simulink model "OMAP"  (R2018b)
settings: Solver=FixedStepDiscrete  StartTime=0.0  StopTime=10.0  FixedStep=0.01  RelTol=1e-3
values from neighbouring files (symbols this model uses):
  Clb_ICADirect_LaneDisp_StateFive = Simulink.Parameter    [omap_ver_442.m]
  Clb_ICADirect_LaneDisp_StateFour = Simulink.Parameter    [omap_ver_442.m]
  Clb_ICADirect_LaneDisp_StateOne = Simulink.Parameter    [omap_ver_442.m]
  Clb_ICADirect_LaneDisp_StateThree = Simulink.Parameter    [omap_ver_442.m]
  Clb_ICADirect_LaneDisp_StateTwo = Simulink.Parameter    [omap_ver_442.m]
  Clb_ICADirect_LaneDisp_StateZero = Simulink.Parameter    [omap_ver_442.m]
  Clb_ICADirect_LaneDispSW = Simulink.Parameter    [omap_ver_442.m]
  Clb_ICADirect_TrnLghtsCom_Switch = Simulink.Parameter    [omap_ver_442.m]
  Clb_ICADirect_TrnLghtsCom_Value = Simulink.Parameter    [omap_ver_442.m]
  Clb_ICADirect_TrnLghtsCrtl_Inhb = Simulink.Parameter    [omap_ver_442.m]
  OMAP_ACCAEB_EMSESC_Decel = Simulink.Parameter    [omap_ver_442.m]
  OMAP_ACCFCW_IC_Decel = Simulink.Parameter    [omap_ver_442.m]
  OMAP_clb_ACC_RVVReqType = Simulink.Parameter    [omap_ver_442.m]
  OMAP_clb_ACC_RVVReqType_Switch = Simulink.Parameter    [omap_ver_442.m]
  OMAP_clb_ACCHeadwayDisplay = Simulink.Parameter    [omap_ver_442.m]
  OMAP_clb_ACCHeadwayDisplay_Switch = Simulink.Parameter    [omap_ver_442.m]
  OMAP_clb_ACCHeadwayIcon = Simulink.Parameter    [omap_ver_442.m]
  OMAP_clb_ACCHeadwayIcon_Switch = Simulink.Parameter    [omap_ver_442.m]
  OMAP_clb_ACCMessagePrompt = Simulink.Parameter    [omap_ver_442.m]
  OMAP_clb_ACCMessagePrompt_Switch = Simulink.Parameter    [omap_ver_442.m]
  OMAP_clb_ACCRequestEPB = Simulink.Parameter    [omap_ver_442.m]
  OMAP_clb_ACCRequestEPB_Switch = Simulink.Parameter    [omap_ver_442.m]
  OMAP_clb_ACCSetSpeed = Simulink.Parameter    [omap_ver_442.m]
  OMAP_clb_ACCSetSpeed_Switch = Simulink.Parameter    [omap_ver_442.m]
  OMAP_clb_ACCSetSpeedDis = Simulink.Parameter    [omap_ver_442.m]
  OMAP_clb_ACCSetSpeedDis_Switch = Simulink.Parameter    [omap_ver_442.m]
  OMAP_clb_ACCState = Simulink.Parameter    [omap_ver_442.m]
  OMAP_clb_ACCState_Switch = Simulink.Parameter    [omap_ver_442.m]
  OMAP_clb_ACCStatusIconDis = Simulink.Parameter    [omap_ver_442.m]
  OMAP_clb_ACCStatusIconDis_Switch = Simulink.Parameter    [omap_ver_442.m]
  OMAP_clb_ACCTorqueReq = Simulink.Parameter    [omap_ver_442.m]
  OMAP_clb_ACCTorqueReq_Switch = Simulink.Parameter    [omap_ver_442.m]
  OMAP_clb_ADAS_State = Simulink.Parameter    [omap_ver_442.m]
  OMAP_clb_ADAS_State_Switch = Simulink.Parameter    [omap_ver_442.m]
  OMAP_clb_AEBAlertReq = Simulink.Parameter    [omap_ver_442.m]
  OMAP_clb_AEBAlertReq_Switch = Simulink.Parameter    [omap_ver_442.m]
  OMAP_clb_AEBBrakingProg = Simulink.Parameter    [omap_ver_442.m]
  OMAP_clb_AEBBrakingProg_Switch = Simulink.Parameter    [omap_ver_442.m]
  OMAP_clb_AEBFaultStatus = Simulink.Parameter    [omap_ver_442.m]
  OMAP_clb_AEBFaultStatus_Switch = Simulink.Parameter    [omap_ver_442.m]
  OMAP_clb_AEBMassageDisp = Simulink.Parameter    [omap_ver_442.m]
  OMAP_clb_AEBMassageDisp_Switch = Simulink.Parameter    [omap_ver_442.m]
  OMAP_clb_AEBState = Simulink.Parameter    [omap_ver_442.m]
  OMAP_clb_AEBState_Switch = Simulink.Parameter    [omap_ver_442.m]
  OMAP_clb_AEBSwitchStatus = Simulink.Parameter    [omap_ver_442.m]
  OMAP_clb_AEBSwitchStatus_Switch = Simulink.Parameter    [omap_ver_442.m]
  OMAP_clb_BrakeRequest = Simulink.Parameter    [omap_ver_442.m]
  OMAP_clb_BrakeRequest_Switch = Simulink.Parameter    [omap_ver_442.m]
  OMAP_clb_DecelerationSet = Simulink.Parameter    [omap_ver_442.m]
  OMAP_clb_DecelerationSet_Switch = Simulink.Parameter    [omap_ver_442.m]
  OMAP_clb_DecelerationType = Simulink.Parameter    [omap_ver_442.m]
  OMAP_clb_DecelerationType_Switch = Simulink.Parameter    [omap_ver_442.m]
  OMAP_clb_DeclControlReq = Simulink.Parameter    [omap_ver_442.m]
  OMAP_clb_DeclControlReq_Switch = Simulink.Parameter    [omap_ver_442.m]
  OMAP_clb_DownorUpGearMinTime = Simulink.Parameter    [omap_ver_442.m]
  OMAP_clb_DownorUpGearMinTime_Switch = Simulink.Parameter    [omap_ver_442.m]
  OMAP_clb_ELKPopupMessage = Simulink.Parameter    [omap_ver_442.m]
  OMAP_clb_ELKPopupMessage_Switch = Simulink.Parameter    [omap_ver_442.m]
  OMAP_clb_ELKSts = Simulink.Parameter    [omap_ver_442.m]
  OMAP_clb_ELKSts_Switch = Simulink.Parameter    [omap_ver_442.m]
  OMAP_clb_ESAFaultSt = Simulink.Parameter    [omap_ver_442.m]
  OMAP_clb_ESAFaultSt_Switch = Simulink.Parameter    [omap_ver_442.m]
  OMAP_clb_ESARequest = Simulink.Parameter    [omap_ver_442.m]
  OMAP_clb_ESARequest_Switch = Simulink.Parameter    [omap_ver_442.m]
  OMAP_clb_ESAState = Simulink.Parameter    [omap_ver_442.m]
  OMAP_clb_ESAState_Switch = Simulink.Parameter    [omap_ver_442.m]
  OMAP_clb_ESATorqueReq = Simulink.Parameter    [omap_ver_442.m]
  OMAP_clb_ESATorqueReq_Switch = Simulink.Parameter    [omap_ver_442.m]
  OMAP_clb_ESCDriveOff = Simulink.Parameter    [omap_ver_442.m]
  OMAP_clb_ESCDriveOff_Switch = Simulink.Parameter    [omap_ver_442.m]
  OMAP_clb_ESCHoldReq = Simulink.Parameter    [omap_ver_442.m]
  OMAP_clb_ESCHoldReq_Switch = Simulink.Parameter    [omap_ver_442.m]
  OMAP_clb_Handsoffwarning = Simulink.Parameter    [omap_ver_442.m]
  OMAP_clb_Handsoffwarning_Switch = Simulink.Parameter    [omap_ver_442.m]
  OMAP_clb_HapticAlarmReq = Simulink.Parameter    [omap_ver_442.m]
  OMAP_clb_HapticAlarmReq_Switch = Simulink.Parameter    [omap_ver_442.m]
  OMAP_clb_HMIPopupMassage = Simulink.Parameter    [omap_ver_442.m]
  OMAP_clb_HMIPopupMassage_Switch = Simulink.Parameter    [omap_ver_442.m]
  OMAP_clb_HWAActionSts = Simulink.Parameter    [omap_ver_442.m]
  OMAP_clb_HWAActionSts_Switch = Simulink.Parameter    [omap_ver_442.m]
  OMAP_clb_HWAMode = Simulink.Parameter    [omap_ver_442.m]
  OMAP_clb_HWAMode_Switch = Simulink.Parameter    [omap_ver_442.m]
  OMAP_clb_HWATurnOnIdctr = Simulink.Parameter    [omap_ver_442.m]
  OMAP_clb_HWATurnOnIdctr_Switch = Simulink.Parameter    [omap_ver_442.m]
  OMAP_clb_ICAMassageDisp = Simulink.Parameter    [omap_ver_442.m]
  OMAP_clb_ICAMassageDisp_Switch = Simulink.Parameter    [omap_ver_442.m]
  OMAP_clb_ICAStatusIcon = Simulink.Parameter    [omap_ver_442.m]
  OMAP_clb_ICAStatusIcon_Switch = Simulink.Parameter    [omap_ver_442.m]
  OMAP_clb_ISLCDriverRemind = Simulink.Parameter    [omap_ver_442.m]
  OMAP_clb_ISLCDriverRemind_Switch = Simulink.Parameter    [omap_ver_442.m]
  OMAP_clb_ISLCState = Simulink.Parameter    [omap_ver_442.m]
  OMAP_clb_ISLCState_Switch = Simulink.Parameter    [omap_ver_442.m]
  OMAP_clb_JAFaultSt = Simulink.Parameter    [omap_ver_442.m]
  OMAP_clb_JAFaultSt_Switch = Simulink.Parameter    [omap_ver_442.m]
  OMAP_clb_LCAPopupMessage = Simulink.Parameter    [omap_ver_442.m]
  OMAP_clb_LCAPopupMessage_Switch = Simulink.Parameter    [omap_ver_442.m]
  OMAP_clb_LCAStatusDisplay = Simulink.Parameter    [omap_ver_442.m]
  OMAP_clb_LCAStatusDisplay_Switch = Simulink.Parameter    [omap_ver_442.m]
  OMAP_clb_LDWStatusDisplay = Simulink.Parameter    [omap_ver_442.m]
  OMAP_clb_LDWStatusDisplay_Switch = Simulink.Parameter    [omap_ver_442.m]
  OMAP_clb_LDWWarningSt = Simulink.Parameter    [omap_ver_442.m]
  OMAP_clb_LDWWarningSt_Switch = Simulink.Parameter    [omap_ver_442.m]
  OMAP_clb_LightControlValid = Simulink.Parameter    [omap_ver_442.m]
  OMAP_clb_LightControlValid_Switch = Simulink.Parameter    [omap_ver_442.m]
  OMAP_clb_LKAActivation = Simulink.Parameter    [omap_ver_442.m]
  OMAP_clb_LKAActivation_Switch = Simulink.Parameter    [omap_ver_442.m]
  OMAP_clb_LKAAngleReq = Simulink.Parameter    [omap_ver_442.m]
  OMAP_clb_LKAAngleReq_Switch = Simulink.Parameter    [omap_ver_442.m]
  OMAP_clb_LKAMode = Simulink.Parameter    [omap_ver_442.m]
  OMAP_clb_LKAMode_Switch = Simulink.Parameter    [omap_ver_442.m]
  OMAP_clb_LKAorELK_CoolTime = Simulink.Parameter    [omap_ver_442.m]
  OMAP_clb_LKAState = Simulink.Parameter    [omap_ver_442.m]
  OMAP_clb_LKAState_Switch = Simulink.Parameter    [omap_ver_442.m]
  OMAP_clb_LKAStatusDisplay = Simulink.Parameter    [omap_ver_442.m]
  OMAP_clb_LKAStatusDisplay_Switch = Simulink.Parameter    [omap_ver_442.m]
  OMAP_clb_LKASwitchState = Simulink.Parameter    [omap_ver_442.m]
  OMAP_clb_LKASwitchState_Switch = Simulink.Parameter    [omap_ver_442.m]
  OMAP_clb_LKATorqFactReq = Simulink.Parameter    [omap_ver_442.m]
  OMAP_clb_LKATorqFactReq_Switch = Simulink.Parameter    [omap_ver_442.m]
  OMAP_clb_PrefillRequest = Simulink.Parameter    [omap_ver_442.m]
  ... (+36 more)
libraries: simulink x184, canmsglib x2
(part 4 of 14)

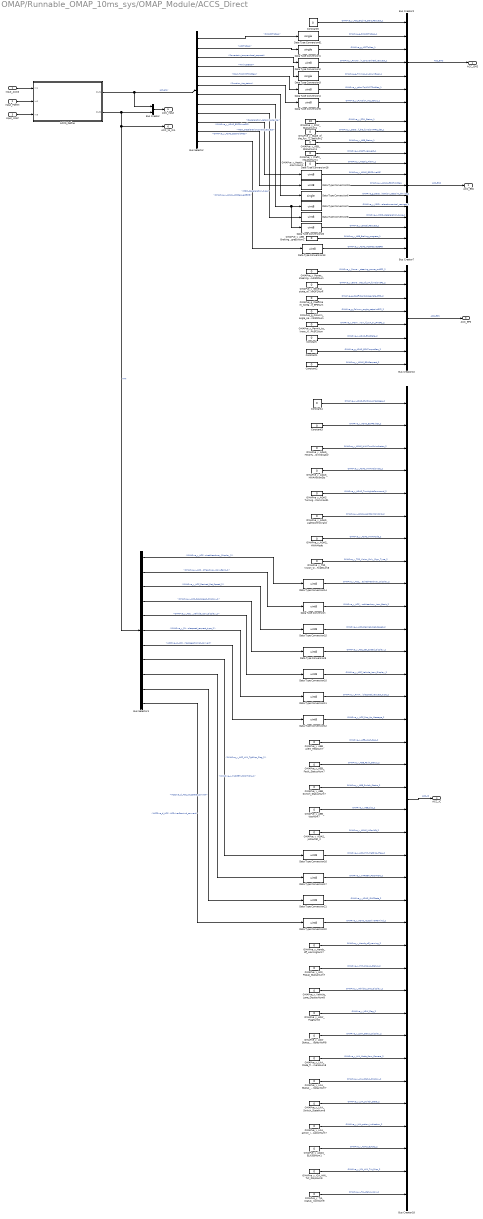
== system OMAP/Runnable_OMAP_10ms_sys/OMAP_Module/ACCS_Direct ==
  Input_ACCS : Inport
  Input_FDMM : Inport  Port=2
  Input_IMAP : Inport  Port=3
  ACCS_Define : Subsystem
  Bus Creator : BusCreator  Inputs=2
  Bus Creator10 : BusCreator  Inputs=8
  Bus Creator18 : BusCreator  Inputs=36
  Bus Creator2 : BusCreator  Inputs=7
  Bus Creator7 : BusCreator  Inputs=13
  Bus Selector : BusSelector  OutputSignals=PotACCTqReq,ACCTqReq,Powertrain_torquewheel_request,TminUpGear,StAcvTqWhlPTPotReq,Function_Acc_status,Deceleration_setpoint_device,MDD_Decelerationcontrol_request,MDD_deceleration_type,OMAPve_y_ADAS_ESCDriveOff,OMAPve_y_ADAS_ESCHoldReq,OMAPve_y_ADAS_ACCRequestEPB
  Bus Selector1 : BusSelector  OutputSignals=OMAPve_y_ACC_DesiredHeadway_Display_2,OMAPve_y_ACC_DesiredHeadway_Icon_Basic_2,OMAPve_y_ACC_Desired_Set_Speed_2,OMAPve_y_ACC_Set_Speed_Display_2,OMAPve_y_ACC_Vehicle_Icon_Display_2,OMAPve_y_RVVACC_Vehiclespeed_request_type_2,ACCSve_d_ACCMessagePrompt_convert,OMAPve_y_ACC_HMI_TgtDisp_Flag_2,OMAPve_y_TARGET_POSITION_2,ACCSve_d_ACC_ISLCState_convert,ACCSve_d_ACC_ISLCDriverRemind_convert
  Constant{,2..5} (5 alike) : Constant  Value=0  OutDataTypeStr=uint8
  Constant1 : Constant  Value=0  OutDataTypeStr=single
  Data Type Conversion{,2,4..5,7..22} (20 alike) : DataTypeConversion  OutDataTypeStr=uint8
  Data Type Conversion{1,3,6,61} (4 alike) : DataTypeConversion  OutDataTypeStr=single
  OMAPve_g_Coefficient_toregulate_EPSNum : Constant  Value=0  OutDataTypeStr=single
  OMAPve_g_Column_angle_setpoint3F2Num : Constant  Value=0  OutDataTypeStr=single
  OMAPve_y_ADAS_ELKStsNum1 : Constant  Value=0  OutDataTypeStr=uint8
  OMAPve_y_ADAS_HWAActionSts : Constant  Value=0  OutDataTypeStr=uint8
  OMAPve_y_ADAS_HWAMode : Constant  Value=0  OutDataTypeStr=uint8
  OMAPve_y_ADAS_HWATurnOnIndicator : Constant  Value=0  OutDataTypeStr=uint8
  OMAPve_y_ADAS_JAFaultSt_2 : Constant  Value=0  OutDataTypeStr=uint8
  OMAPve_y_ADAS_LightControlValid : Constant  Value=0  OutDataTypeStr=uint8
  OMAPve_y_ADAS_TurnLightsCommand1 : Constant  Value=0  OutDataTypeStr=uint8
  OMAPve_y_AEB_Alert_ReqNum7 : Constant  Value=0  OutDataTypeStr=uint8
  OMAPve_y_AEB_Braking_progressNum1 : Constant  Value=0  OutDataTypeStr=uint8
  OMAPve_y_AEB_Fault_StatusNum7 : Constant  Value=0  OutDataTypeStr=uint8
  OMAPve_y_AEB_StatusNum1 : Constant  Value=0  OutDataTypeStr=uint8
  OMAPve_y_AEB_Switch_StatusNum7 : Constant  Value=0  OutDataTypeStr=uint8
  OMAPve_y_AEB_tipsNum7 : Constant  Value=0  OutDataTypeStr=uint8
  OMAPve_y_FCW_StatusNum1 : Constant  Value=10  OutDataTypeStr=uint8
  OMAPve_y_General_state_of_LKA_function3F2Num : Constant  Value=0  OutDataTypeStr=uint8
  OMAPve_y_HMI_Popup_StatusNum7 : Constant  Value=0  OutDataTypeStr=uint8
  OMAPve_y_Hands_off_warningNum7 : Constant  Value=0  OutDataTypeStr=uint8
  OMAPve_y_Haptic_AlarmNum1 : Constant  Value=0  OutDataTypeStr=uint8
  OMAPve_y_ICA_HMI_Txt_DispNum9 : Constant  Value=0  OutDataTypeStr=uint8
  OMAPve_y_LDW_FlagNum8 : Constant  Value=0  OutDataTypeStr=uint8
  OMAPve_y_LDW_Status_DisplayNum8 : Constant  Value=0  OutDataTypeStr=uint8
  OMAPve_y_LKA_Mode_from_CameraNum8 : Constant  Value=0  OutDataTypeStr=uint8
  OMAPve_y_LKA_Status_DisplayNum7 : Constant  Value=0  OutDataTypeStr=uint8
  OMAPve_y_LKA_Switch_StateNum8 : Constant  Value=0  OutDataTypeStr=uint8
  OMAPve_y_LKA_action_indicationNum7 : Constant  Value=0  OutDataTypeStr=uint8
  OMAPve_y_Permit_to_know_if_LKA_or_LPA3F2Num : Constant  Value=0  OutDataTypeStr=uint8
  OMAPve_y_Power_steering_power_cut3F2Num : Constant  Value=0  OutDataTypeStr=uint8
  OMAPve_y_Prefill_requestNum1 : Constant  Value=0  OutDataTypeStr=uint8
  OMAPve_y_State_of_the_functionFARC_detNum1 : Constant  Value=0  OutDataTypeStr=uint8
  OMAPve_y_TJA_status_iconNum9 : Constant  Value=0  OutDataTypeStr=uint8
  OMAPve_y_TSR_Vision_Only_Sign_TypeNum8 : Constant  Value=0  OutDataTypeStr=uint8
  OMAPve_y_Vehicle_Lane_DisplayNum8 : Constant  Value=0  OutDataTypeStr=uint8
  ACC_EMS : Outport
  ACC_ESC : Outport  Port=2
  ACC_EPS : Outport  Port=3
  ACC_IC : Outport  Port=4
  ACC_Input : Outport  Port=5
  ACC_to_ICA : Outport  Port=6
  wires:
  Bus Selector/9 -> Data Type Conversion8/1  "<MDD_deceleration_type>"
  Bus Selector/8 -> Data Type Conversion20/1, Data Type Conversion7/1  "<MDD_Decelerationcontrol_request>"
  Bus Selector/7 -> Data Type Conversion6/1  "<Deceleration_setpoint_device>"
  Bus Selector/6 -> Data Type Conversion5/1  "<Function_Acc_status>"
  Bus Selector/5 -> Data Type Conversion4/1  "<StAcvTqWhlPTPotReq>"
  Bus Selector/4 -> Data Type Conversion3/1  "<TminUpGear>"
  Bus Selector/3 -> Data Type Conversion2/1  "<Powertrain_torquewheel_request>"
  Bus Selector/2 -> Data Type Conversion1/1  "<ACCTqReq>"
  Bus Selector/1 -> Data Type Conversion61/1  "<PotACCTqReq>"
  Input_FDMM/1 -> ACCS_Define/2(In2)
  Input_ACCS/1 -> ACCS_Define/1(In1)
  Bus Selector1/6 -> Data Type Conversion11/1  "<OMAPve_y_RVVACC_Vehiclespeed_request_type_2>"
  Bus Selector1/7 -> Data Type Conversion12/1  "<ACCSve_d_ACCMessagePrompt_convert>"
  Data Type Conversion1/1 -> Bus Creator2/3  "OMAPve_g_ACCTqReq_1"
  OMAPve_y_AEB_StatusNum1/1 -> Bus Creator7/3  "OMAPve_y_AEB_Status_1"
  Data Type Conversion6/1 -> Bus Creator7/8  "OMAPve_g_Deceleration_setpoint_device_1"
  Data Type Conversion8/1 -> Bus Creator7/10  "OMAPve_y_MDD_deceleration_type_1"
  Bus Selector1/5 -> Data Type Conversion10/1  "<OMAPve_y_ACC_Vehicle_Icon_Display_2>"
  Bus Creator18/1 -> ACC_IC/1  "ACC_IC"
  OMAPve_y_LDW_Status_DisplayNum8/1 -> Bus Creator18/29  "OMAPve_y_LDW_Status_Display_2"
  Bus Creator7/1 -> ACC_ESC/1  "ACC_ESC"
  OMAPve_y_AEB_tipsNum7/1 -> Bus Creator18/19  "OMAPve_y_AEB_tips_2"
  Bus Selector1/9 -> Data Type Conversion17/1  "<OMAPve_y_TARGET_POSITION_2>"
  Bus Selector1/3 -> Data Type Conversion15/1  "<OMAPve_y_ACC_Desired_Set_Speed_2>"
  Bus Selector1/1 -> Data Type Conversion14/1  "<OMAPve_y_ACC_DesiredHeadway_Display_2>"
  OMAPve_y_HMI_Popup_StatusNum7/1 -> Bus Creator18/26  "OMAPve_y_HMI_Popup_Status_2"
  OMAPve_y_AEB_Alert_ReqNum7/1 -> Bus Creator18/16  "OMAPve_y_AEB_Alert_Req_2"
  Bus Creator2/1 -> ACC_EMS/1  "ACC_EMS"
  OMAPve_y_TSR_Vision_Only_Sign_TypeNum8/1 -> Bus Creator18/8  "OMAPve_y_TSR_Vision_Only_Sign_Type_2"
  OMAPve_y_LDW_FlagNum8/1 -> Bus Creator18/28  "OMAPve_y_LDW_Flag_2"
  OMAPve_y_AEB_Fault_StatusNum7/1 -> Bus Creator18/17  "OMAPve_y_AEB_Fault_Status_2"
  OMAPve_y_State_of_the_functionFARC_detNum1/1 -> Bus Creator7/2  "OMAPve_y_State_of_the_functionFARC_det_1"
  OMAPve_y_Haptic_AlarmNum1/1 -> Bus Creator7/5  "OMAPve_y_Haptic_Alarm_1"
  OMAPve_y_ICA_HMI_Txt_DispNum9/1 -> Bus Creator18/35  "OMAPve_y_ICA_HMI_Txt_Disp_2"
  Data Type Conversion4/1 -> Bus Creator2/6  "OMAPve_y_stAcvTqWhlPTPotReq_1"
  Data Type Conversion20/1 -> Bus Creator7/11  "OMAPve_y_Decel_Request_1"
  Bus Selector1/2 -> Data Type Conversion/1  "<OMAPve_y_ACC_DesiredHeadway_Icon_Basic_2>"
  Data Type Conversion61/1 -> Bus Creator2/2  "OMAPve_g_PotACCTqReq_1"
  Bus Selector1/8 -> Data Type Conversion16/1  "<OMAPve_y_ACC_HMI_TgtDisp_Flag_2>"
  OMAPve_y_FCW_StatusNum1/1 -> Bus Creator7/1  "OMAPve_y_FCW_Status_1"
  OMAPve_y_Hands_off_warningNum7/1 -> Bus Creator18/25  "OMAPve_y_Hands_off_warning_2"
  OMAPve_y_AEB_Braking_progressNum1/1 -> Bus Creator7/12  "OMAPve_y_AEB_Braking_progress_1"
  Data Type Conversion5/1 -> Bus Creator2/7  "OMAPve_y_Function_Acc_status_1"
  OMAPve_y_LKA_Status_DisplayNum7/1 -> Bus Creator18/31  "OMAPve_y_LKA_Status_Display_2"
  Data Type Conversion3/1 -> Bus Creator2/5  "OMAPve_g_TminUp_or_downGear_1"
  OMAPve_y_Vehicle_Lane_DisplayNum8/1 -> Bus Creator18/27  "OMAPve_y_Vehicle_Lane_Display_2"
  OMAPve_y_AEB_Switch_StatusNum7/1 -> Bus Creator18/18  "OMAPve_y_AEB_Switch_Status_2"
  Constant5/1 -> Bus Creator2/1  "OMAPve_y_ACC_Engine_Start_Request_1"
  OMAPve_y_TJA_status_iconNum9/1 -> Bus Creator18/36  "OMAPve_y_TJA_status_icon_2"
  OMAPve_y_LKA_action_indicationNum7/1 -> Bus Creator18/33  "OMAPve_y_LKA_action_indication_2"
  Bus Selector1/4 -> Data Type Conversion9/1  "<OMAPve_y_ACC_Set_Speed_Display_2>"
  OMAPve_y_Prefill_requestNum1/1 -> Bus Creator7/4  "OMAPve_y_Prefill_request_1"
  Data Type Conversion7/1 -> Bus Creator7/9  "OMAPve_y_MDD_Decelerationcontrol_request_1"
  OMAPve_y_LKA_Switch_StateNum8/1 -> Bus Creator18/32  "OMAPve_y_LKA_Switch_State_2"
  Data Type Conversion2/1 -> Bus Creator2/4  "OMAPve_y_Powertrain_torquewheel_request_1"
  OMAPve_y_LKA_Mode_from_CameraNum8/1 -> Bus Creator18/30  "OMAPve_y_LKA_Mode_from_Camera_2"
  ACCS_Define/1(Out1) -> Bus Creator/1, Bus Selector/1  "actuator"
  OMAPve_y_Power_steering_power_cut3F2Num/1 -> Bus Creator10/1  "OMAPve_y_Power_steering_power_cut3F2_2"
  OMAPve_g_Coefficient_toregulate_EPSNum/1 -> Bus Creator10/3  "OMAPve_g_Coefficient_toregulate_EPS_2"
  OMAPve_y_Permit_to_know_if_LKA_or_LPA3F2Num/1 -> Bus Creator10/5  "OMAPve_y_Permit_to_know_if_LKA_or_LPA3F2_2"
  Bus Creator10/1 -> ACC_EPS/1  "ACC_EPS"
  OMAPve_y_General_state_of_LKA_function3F2Num/1 -> Bus Creator10/2  "OMAPve_y_General_state_of_LKA_function3F2_2"
  OMAPve_g_Column_angle_setpoint3F2Num/1 -> Bus Creator10/4  "OMAPve_g_Column_angle_setpoint3F2_2"
  Input_IMAP/1 -> ACCS_Define/3(In3)
  ACCS_Define/2(Out2) -> ACC_to_ICA/1, Bus Selector1/1, Bus Creator/2  "HMI"
  Bus Creator/1 -> ACC_Input/1
  Data Type Conversion/1 -> Bus Creator18/10  "OMAPve_y_ACC_DesiredHeadway_Icon_Basic_2"
  Data Type Conversion9/1 -> Bus Creator18/12  "OMAPve_y_ACC_Set_Speed_Display_2"
  Data Type Conversion10/1 -> Bus Creator18/13  "OMAPve_y_ACC_Vehicle_Icon_Display_2"
  Data Type Conversion11/1 -> Bus Creator18/14  "OMAPve_y_RVVACC_Vehiclespeed_request_type_2"
  Data Type Conversion12/1 -> Bus Creator18/15  "OMAPve_y_ACC_Pop_Up_Message_2"
  Data Type Conversion14/1 -> Bus Creator18/9  "OMAPve_y_ACC_DesiredHeadway_Display_2"
  Data Type Conversion15/1 -> Bus Creator18/11  "OMAPve_y_ACC_Desired_Set_Speed_2"
  Data Type Conversion16/1 -> Bus Creator18/21  "OMAPve_y_ACC_HMI_TgtDisp_Flag_2"
  Data Type Conversion17/1 -> Bus Creator18/22  "OMAPve_y_TARGET_POSITION_2"
  OMAPve_y_ADAS_ELKStsNum1/1 -> Bus Creator18/34  "OMAPve_y_ADAS_ELKSts_2"
  Data Type Conversion19/1 -> Bus Creator7/7  "OMAPve_y_ADAS_ESCHoldReq"
  Data Type Conversion18/1 -> Bus Creator7/6  "OMAPve_y_ADAS_ESCDriveOff"
  Bus Selector/10 -> Data Type Conversion18/1  "<OMAPve_y_ADAS_ESCDriveOff>"
  Bus Selector/11 -> Data Type Conversion19/1  "<OMAPve_y_ADAS_ESCHoldReq>"
  Data Type Conversion13/1 -> Bus Creator7/13  "OMAPve_y_ADAS_ACCRequestEPB"
  Bus Selector/12 -> Data Type Conversion13/1  "<OMAPve_y_ADAS_ACCRequestEPB>"
  OMAPve_y_ADAS_JAFaultSt_2/1 -> Bus Creator18/20  "OMAPve_y_ADAS_JAFaultSt_2"
  Bus Selector1/10 -> Data Type Conversion21/1  "<ACCSve_d_ACC_ISLCState_convert>"
  Bus Selector1/11 -> Data Type Conversion22/1  "<ACCSve_d_ACC_ISLCDriverRemind_convert>"
  Data Type Conversion21/1 -> Bus Creator18/23  "OMAPve_y_ADAS_ISLCState_2"
  Data Type Conversion22/1 -> Bus Creator18/24  "OMAPve_y_ADAS_ISLCDriverRemind_2"
  OMAPve_y_ADAS_LightControlValid/1 -> Bus Creator18/6  "OMAPve_y_ADAS_LightControlValid_2"
  OMAPve_y_ADAS_HWAActionSts/1 -> Bus Creator18/4  "OMAPve_y_ADAS_HWAActionSts_2"
  OMAPve_y_ADAS_HWATurnOnIndicator/1 -> Bus Creator18/3  "OMAPve_y_ADAS_HWATurnOnIndicator_2"
  OMAPve_y_ADAS_HWAMode/1 -> Bus Creator18/7  "OMAPve_y_ADAS_HWAMode_2"
  OMAPve_y_ADAS_TurnLightsCommand1/1 -> Bus Creator18/5  "OMAPve_y_ADAS_TurnLightsCommand_2"
  Constant2/1 -> Bus Creator10/8  "OMAPve_y_ADAS_ESARequest_2"
  Constant/1 -> Bus Creator10/6  "OMAPve_y_ADAS_ESAState_2"
  Constant1/1 -> Bus Creator10/7  "OMAPve_g_ADAS_ESATorqueReq_2"
  Constant3/1 -> Bus Creator18/2  "OMAPve_y_ADAS_ESAFaultSt_2"
  Constant4/1 -> Bus Creator18/1  "OMAPve_y_ADAS_ELKPopupMessage_2"

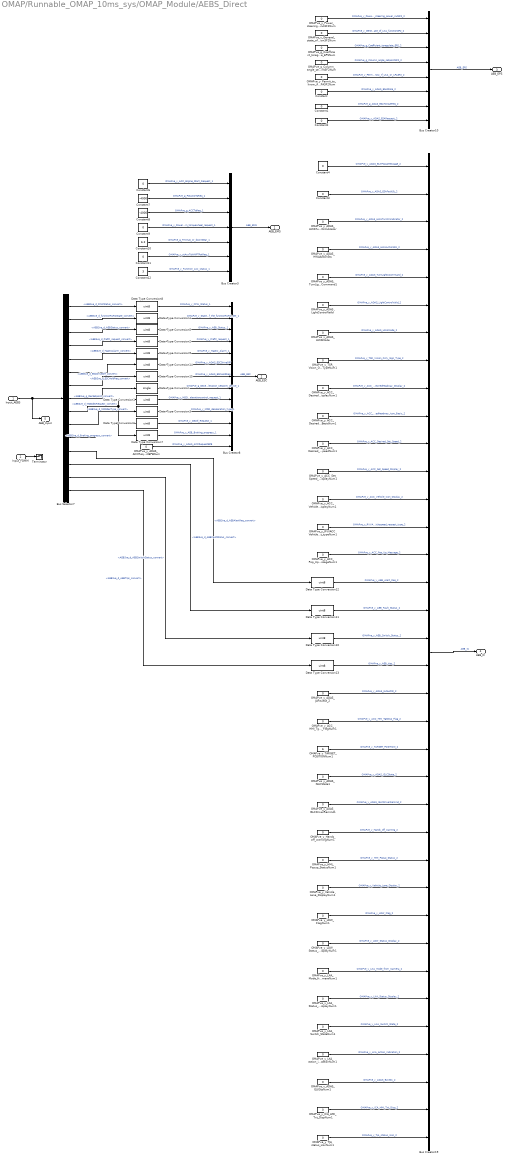
== system OMAP/Runnable_OMAP_10ms_sys/OMAP_Module/AEBS_Direct ==
  Input_AEBS : Inport
  Input_FDMM : Inport  Port=2
  Bus Creator10 : BusCreator  Inputs=8
  Bus Creator19 : BusCreator  Inputs=36
  Bus Creator3 : BusCreator  Inputs=7
  Bus Creator8 : BusCreator  Inputs=13
  Bus Selector7 : BusSelector  OutputSignals=AEBSve_d_FCWStatus_convert,AEBSve_d_functionFARCState_convert,AEBSve_d_AEBStatus_convert,AEBSve_d_Prefill_request_convert,AEBSve_d_HapticAlarm_convert,AEBSve_d_ESCDriveOff_convert,AEBSve_d_ESCHoldReq_convert,AEBSve_g_DecSetpoint_convert,AEBSve_d_MDDdecRequest_convert,AEBSve_d_MDDdecType_convert,AEBSve_d_Braking_progress_convert,AEBSve_d_AEBAlertReq_convert,AEBSve_d_AEBFaultStatus_convert,AEBSve_d_AEBSwitchStatus_convert,AEBSve_d_AEBTips_convert
  Constant{,2..4,6,9,11} (7 alike) : Constant  Value=0  OutDataTypeStr=uint8
  Constant1 : Constant  Value=0  OutDataTypeStr=single
  Constant10 : Constant  Value=6.2  OutDataTypeStr=single
  Constant12 : Constant  Value=3  OutDataTypeStr=uint8
  Constant7 : Constant  Value=-4000  OutDataTypeStr=single
  Constant8 : Constant  Value=-4000  OutDataTypeStr=single
  Data Type Conversion : DataTypeConversion  OutDataTypeStr=single
  Data Type Conversion{1..15} (15 alike) : DataTypeConversion  OutDataTypeStr=uint8
  OMAPve_g_Coefficient_toregulate_EPSNum : Constant  Value=0  OutDataTypeStr=single
  OMAPve_g_Column_angle_setpoint3F2Num : Constant  Value=0  OutDataTypeStr=single
  OMAPve_y_ACC_DesiredHeadway_DisplayNum1 : Constant  Value=0  OutDataTypeStr=uint8
  OMAPve_y_ACC_DesiredHeadway_Icon_BasicNum1 : Constant  Value=0  OutDataTypeStr=uint8
  OMAPve_y_ACC_Desired_Set_SpeedNum1 : Constant  Value=0  OutDataTypeStr=uint8
  OMAPve_y_ACC_HMI_TgtDisp_FlagNum1 : Constant  Value=0  OutDataTypeStr=uint8
  OMAPve_y_ACC_Pop_Up_MessageNum1 : Constant  Value=0  OutDataTypeStr=uint8
  OMAPve_y_ACC_Set_Speed_DisplayNum1 : Constant  Value=0  OutDataTypeStr=uint8
  OMAPve_y_ACC_Vehicle_Icon_DisplayNum1 : Constant  Value=0  OutDataTypeStr=uint8
  OMAPve_y_ADAS_ACCRequestEPBNum : Constant  Value=0  OutDataTypeStr=uint8
  OMAPve_y_ADAS_ELKStsNum1 : Constant  Value=0  OutDataTypeStr=uint8
  OMAPve_y_ADAS_HWAActionSts : Constant  Value=0  OutDataTypeStr=uint8
  OMAPve_y_ADAS_HWAMode : Constant  Value=0  OutDataTypeStr=uint8
  OMAPve_y_ADAS_HWATurnOnIndicator : Constant  Value=0  OutDataTypeStr=uint8
  OMAPve_y_ADAS_ISLCDriverRemind1 : Constant  Value=0  OutDataTypeStr=uint8
  OMAPve_y_ADAS_ISLCState1 : Constant  Value=0  OutDataTypeStr=uint8
  OMAPve_y_ADAS_JAFaultSt_2 : Constant  Value=0  OutDataTypeStr=uint8
  OMAPve_y_ADAS_LightControlValid : Constant  Value=0  OutDataTypeStr=uint8
  OMAPve_y_ADAS_TurnLightsCommand1 : Constant  Value=0  OutDataTypeStr=uint8
  OMAPve_y_General_state_of_LKA_function3F2Num : Constant  Value=0  OutDataTypeStr=uint8
  OMAPve_y_HMI_Popup_StatusNum1 : Constant  Value=0  OutDataTypeStr=uint8
  OMAPve_y_Hands_off_warningNum1 : Constant  Value=0  OutDataTypeStr=uint8
  OMAPve_y_ICA_HMI_Txt_DispNum1 : Constant  Value=0  OutDataTypeStr=uint8
  OMAPve_y_LDW_FlagNum1 : Constant  Value=0  OutDataTypeStr=uint8
  OMAPve_y_LDW_Status_DisplayNum1 : Constant  Value=0  OutDataTypeStr=uint8
  OMAPve_y_LKA_Mode_from_CameraNum1 : Constant  Value=0  OutDataTypeStr=uint8
  OMAPve_y_LKA_Status_DisplayNum1 : Constant  Value=0  OutDataTypeStr=uint8
  OMAPve_y_LKA_Switch_StateNum1 : Constant  Value=0  OutDataTypeStr=uint8
  OMAPve_y_LKA_action_indicationNum1 : Constant  Value=0  OutDataTypeStr=uint8
  OMAPve_y_Permit_to_know_if_LKA_or_LPA3F2Num : Constant  Value=0  OutDataTypeStr=uint8
  OMAPve_y_Power_steering_power_cut3F2Num : Constant  Value=0  OutDataTypeStr=uint8
  OMAPve_y_RVVACC_Vehiclespeed_request_typeNum1 : Constant  Value=0  OutDataTypeStr=uint8
  OMAPve_y_TARGET_POSITIONNum1 : Constant  Value=6  OutDataTypeStr=uint8
  OMAPve_y_TJA_status_iconNum1 : Constant  Value=0  OutDataTypeStr=uint8
  OMAPve_y_TSR_Vision_Only_Sign_TypeNum1 : Constant  Value=0  OutDataTypeStr=uint8
  OMAPve_y_Vehicle_Lane_DisplayNum1 : Constant  Value=0  OutDataTypeStr=uint8
  Terminator : Terminator
  AEB_EMS : Outport
  AEB_ESC : Outport  Port=2
  AEB_EPS : Outport  Port=3
  AEB_IC : Outport  Port=4
  AEB_Input : Outport  Port=5
  wires:
  OMAPve_y_LDW_FlagNum1/1 -> Bus Creator19/28  "OMAPve_y_LDW_Flag_2"
  Bus Selector7/15 -> Data Type Conversion13/1  "<AEBSve_d_AEBTips_convert>"
  OMAPve_y_Vehicle_Lane_DisplayNum1/1 -> Bus Creator19/27  "OMAPve_y_Vehicle_Lane_Display_2"
  Bus Selector7/1 -> Data Type Conversion8/1  "<AEBSve_d_FCWStatus_convert>"
  Bus Selector7/8 -> Data Type Conversion/1  "<AEBSve_g_DecSetpoint_convert>"
  OMAPve_y_ACC_DesiredHeadway_DisplayNum1/1 -> Bus Creator19/9  "OMAPve_y_ACC_DesiredHeadway_Display_2"
  Data Type Conversion13/1 -> Bus Creator19/19  "OMAPve_y_AEB_tips_2"
  OMAPve_y_HMI_Popup_StatusNum1/1 -> Bus Creator19/26  "OMAPve_y_HMI_Popup_Status_2"
  OMAPve_y_Hands_off_warningNum1/1 -> Bus Creator19/25  "OMAPve_y_Hands_off_warning_2"
  Bus Creator3/1 -> AEB_EMS/1  "AEB_EMS"
  OMAPve_y_ACC_DesiredHeadway_Icon_BasicNum1/1 -> Bus Creator19/10  "OMAPve_y_ACC_DesiredHeadway_Icon_Basic_2"
  Constant9/1 -> Bus Creator3/4  "OMAPve_y_Powertrain_torquewheel_request_1"
  OMAPve_y_ACC_Vehicle_Icon_DisplayNum1/1 -> Bus Creator19/13  "OMAPve_y_ACC_Vehicle_Icon_Display_2"
  Data Type Conversion9/1 -> Bus Creator8/5  "OMAPve_y_Haptic_Alarm_1"
  Data Type Conversion2/1 -> Bus Creator8/4  "OMAPve_y_Prefill_request_1"
  Bus Selector7/13 -> Data Type Conversion11/1  "<AEBSve_d_AEBFaultStatus_convert>"
  OMAPve_y_LKA_Switch_StateNum1/1 -> Bus Creator19/32  "OMAPve_y_LKA_Switch_State_2"
  Bus Selector7/3 -> Data Type Conversion5/1  "<AEBSve_d_AEBStatus_convert>"
  Bus Selector7/2 -> Data Type Conversion4/1  "<AEBSve_d_functionFARCState_convert>"
  Data Type Conversion10/1 -> Bus Creator19/18  "OMAPve_y_AEB_Switch_Status_2"
  OMAPve_y_TARGET_POSITIONNum1/1 -> Bus Creator19/22  "OMAPve_y_TARGET_POSITION_2"
  Bus Selector7/4 -> Data Type Conversion2/1  "<AEBSve_d_Prefill_request_convert>"
  OMAPve_y_RVVACC_Vehiclespeed_request_typeNum1/1 -> Bus Creator19/14  "OMAPve_y_RVVACC_Vehiclespeed_request_type_2"
  Input_AEBS/1 -> Bus Selector7/1, AEB_Input/1
  Bus Selector7/12 -> Data Type Conversion12/1  "<AEBSve_d_AEBAlertReq_convert>"
  Bus Creator19/1 -> AEB_IC/1  "AEB_IC"
  Bus Creator8/1 -> AEB_ESC/1  "AEB_ESC"
  OMAPve_y_LDW_Status_DisplayNum1/1 -> Bus Creator19/29  "OMAPve_y_LDW_Status_Display_2"
  Bus Selector7/10 -> Data Type Conversion3/1  "<AEBSve_d_MDDdecType_convert>"
  OMAPve_y_ACC_Set_Speed_DisplayNum1/1 -> Bus Creator19/12  "OMAPve_y_ACC_Set_Speed_Display_2"
  OMAPve_y_LKA_Mode_from_CameraNum1/1 -> Bus Creator19/30  "OMAPve_y_LKA_Mode_from_Camera_2"
  Bus Selector7/14 -> Data Type Conversion10/1  "<AEBSve_d_AEBSwitchStatus_convert>"
  Data Type Conversion12/1 -> Bus Creator19/16  "OMAPve_y_AEB_Alert_Req_2"
  OMAPve_y_ACC_Desired_Set_SpeedNum1/1 -> Bus Creator19/11  "OMAPve_y_ACC_Desired_Set_Speed_2"
  Data Type Conversion7/1 -> Bus Creator8/12  "OMAPve_y_AEB_Braking_progress_1"
  Data Type Conversion11/1 -> Bus Creator19/17  "OMAPve_y_AEB_Fault_Status_2"
  OMAPve_y_ICA_HMI_Txt_DispNum1/1 -> Bus Creator19/35  "OMAPve_y_ICA_HMI_Txt_Disp_2"
  OMAPve_y_ACC_Pop_Up_MessageNum1/1 -> Bus Creator19/15  "OMAPve_y_ACC_Pop_Up_Message_2"
  Data Type Conversion6/1 -> Bus Creator8/11  "OMAPve_y_Decel_Request_1"
  OMAPve_y_LKA_action_indicationNum1/1 -> Bus Creator19/33  "OMAPve_y_LKA_action_indication_2"
  Constant12/1 -> Bus Creator3/7  "OMAPve_y_Function_Acc_status_1"
  OMAPve_y_LKA_Status_DisplayNum1/1 -> Bus Creator19/31  "OMAPve_y_LKA_Status_Display_2"
  Data Type Conversion4/1 -> Bus Creator8/2  "OMAPve_y_State_of_the_functionFARC_det_1"
  Data Type Conversion5/1 -> Bus Creator8/3  "OMAPve_y_AEB_Status_1"
  OMAPve_y_TJA_status_iconNum1/1 -> Bus Creator19/36  "OMAPve_y_TJA_status_icon_2"
  Data Type Conversion8/1 -> Bus Creator8/1  "OMAPve_y_FCW_Status_1"
  OMAPve_y_ACC_HMI_TgtDisp_FlagNum1/1 -> Bus Creator19/21  "OMAPve_y_ACC_HMI_TgtDisp_Flag_2"
  OMAPve_y_TSR_Vision_Only_Sign_TypeNum1/1 -> Bus Creator19/8  "OMAPve_y_TSR_Vision_Only_Sign_Type_2"
  Data Type Conversion3/1 -> Bus Creator8/10  "OMAPve_y_MDD_deceleration_type_1"
  Bus Selector7/5 -> Data Type Conversion9/1  "<AEBSve_d_HapticAlarm_convert>"
  Constant11/1 -> Bus Creator3/6  "OMAPve_y_stAcvTqWhlPTPotReq_1"
  Constant8/1 -> Bus Creator3/3  "OMAPve_g_ACCTqReq_1"
  Constant10/1 -> Bus Creator3/5  "OMAPve_g_TminUp_or_downGear_1"
  Constant6/1 -> Bus Creator3/1  "OMAPve_y_ACC_Engine_Start_Request_1"
  Constant7/1 -> Bus Creator3/2  "OMAPve_g_PotACCTqReq_1"
  Bus Selector7/9 -> Data Type Conversion7/1, Data Type Conversion6/1, Data Type Conversion1/1  "<AEBSve_d_MDDdecRequest_convert>"
  Data Type Conversion/1 -> Bus Creator8/8  "OMAPve_g_Deceleration_setpoint_device_1"
  Data Type Conversion1/1 -> Bus Creator8/9  "OMAPve_y_MDD_Decelerationcontrol_request_1"
  OMAPve_g_Coefficient_toregulate_EPSNum/1 -> Bus Creator10/3  "OMAPve_g_Coefficient_toregulate_EPS_2"
  OMAPve_y_Power_steering_power_cut3F2Num/1 -> Bus Creator10/1  "OMAPve_y_Power_steering_power_cut3F2_2"
  OMAPve_y_General_state_of_LKA_function3F2Num/1 -> Bus Creator10/2  "OMAPve_y_General_state_of_LKA_function3F2_2"
  Bus Creator10/1 -> AEB_EPS/1  "AEB_EPS"
  OMAPve_y_Permit_to_know_if_LKA_or_LPA3F2Num/1 -> Bus Creator10/5  "OMAPve_y_Permit_to_know_if_LKA_or_LPA3F2_2"
  OMAPve_g_Column_angle_setpoint3F2Num/1 -> Bus Creator10/4  "OMAPve_g_Column_angle_setpoint3F2_2"
  Input_FDMM/1 -> Terminator/1
  OMAPve_y_ADAS_ELKStsNum1/1 -> Bus Creator19/34  "OMAPve_y_ADAS_ELKSts_2"
  Data Type Conversion14/1 -> Bus Creator8/6  "OMAPve_y_ADAS_ESCDriveOff"
  Data Type Conversion15/1 -> Bus Creator8/7  "OMAPve_y_ADAS_ESCHoldReq"
  Bus Selector7/6 -> Data Type Conversion14/1  "<AEBSve_d_ESCDriveOff_convert>"
  Bus Selector7/7 -> Data Type Conversion15/1  "<AEBSve_d_ESCHoldReq_convert>"
  OMAPve_y_ADAS_ACCRequestEPBNum/1 -> Bus Creator8/13  "OMAPve_y_ADAS_ACCRequestEPB"
  OMAPve_y_ADAS_JAFaultSt_2/1 -> Bus Creator19/20  "OMAPve_y_ADAS_JAFaultSt_2"
  Bus Selector7/11 -> ?  "<AEBSve_d_Braking_progress_convert>"
  OMAPve_y_ADAS_ISLCState1/1 -> Bus Creator19/23  "OMAPve_y_ADAS_ISLCState_2"
  OMAPve_y_ADAS_ISLCDriverRemind1/1 -> Bus Creator19/24  "OMAPve_y_ADAS_ISLCDriverRemind_2"
  OMAPve_y_ADAS_LightControlValid/1 -> Bus Creator19/6  "OMAPve_y_ADAS_LightControlValid_2"
  OMAPve_y_ADAS_HWAActionSts/1 -> Bus Creator19/4  "OMAPve_y_ADAS_HWAActionSts_2"
  OMAPve_y_ADAS_HWATurnOnIndicator/1 -> Bus Creator19/3  "OMAPve_y_ADAS_HWATurnOnIndicator_2"
  OMAPve_y_ADAS_HWAMode/1 -> Bus Creator19/7  "OMAPve_y_ADAS_HWAMode_2"
  OMAPve_y_ADAS_TurnLightsCommand1/1 -> Bus Creator19/5  "OMAPve_y_ADAS_TurnLightsCommand_2"
  Constant1/1 -> Bus Creator10/7  "OMAPve_g_ADAS_ESATorqueReq_2"
  Constant/1 -> Bus Creator10/6  "OMAPve_y_ADAS_ESAState_2"
  Constant2/1 -> Bus Creator10/8  "OMAPve_y_ADAS_ESARequest_2"
  Constant3/1 -> Bus Creator19/2  "OMAPve_y_ADAS_ESAFaultSt_2"
  Constant4/1 -> Bus Creator19/1  "OMAPve_y_ADAS_ELKPopupMessage_2"

== system OMAP/Runnable_OMAP_10ms_sys/OMAP_Module/Calib ==
  Bus Creator : BusCreator  Inputs=58
  Constant : Constant  Value=OMAP_clb_ACCTorqueReq_Switch
  Constant1 : Constant  Value=OMAP_clb_TorqueActivReq_Switch
  Constant10 : Constant  Value=OMAP_clb_AEBState_Switch
  Constant11 : Constant  Value=OMAP_clb_BrakeRequest_Switch
  Constant12 : Constant  Value=OMAP_clb_AEBBrakingProg_Switch
  Constant13 : Constant  Value=OMAP_clb_HapticAlarmReq_Switch
  Constant14 : Constant  Value=OMAP_clb_ACCRequestEPB_Switch
  Constant15 : Constant  Value=OMAP_clb_LKAState_Switch
  Constant16 : Constant  Value=OMAP_clb_LKATorqFactReq_Switch
  Constant17 : Constant  Value=OMAP_clb_LKAAngleReq_Switch
  Constant18 : Constant  Value=OMAP_clb_LKAActivation_Switch
  Constant19 : Constant  Value=OMAP_clb_ESAState_Switch
  Constant2 : Constant  Value=OMAP_clb_DownorUpGearMinTime_Switch
  Constant20 : Constant  Value=OMAP_clb_ESATorqueReq_Switch
  Constant21 : Constant  Value=OMAP_clb_ESARequest_Switch
  Constant22 : Constant  Value=OMAP_clb_UpDownGearChange_Switch
  Constant23 : Constant  Value=OMAP_clb_ELKPopupMessage_Switch
  Constant24 : Constant  Value=OMAP_clb_ESAFaultSt_Switch
  Constant25 : Constant  Value=OMAP_clb_HWAMode_Switch
  Constant26 : Constant  Value=OMAP_clb_HWATurnOnIdctr_Switch
  Constant27 : Constant  Value=OMAP_clb_HWAActionSts_Switch
  Constant28 : Constant  Value=OMAP_clb_LightControlValid_Switch
  Constant29 : Constant  Value=OMAP_clb_ISLCState_Switch
  Constant3 : Constant  Value=OMAP_clb_ACCState_Switch
  Constant30 : Constant  Value=OMAP_clb_ISLCDriverRemind_Switch
  Constant31 : Constant  Value=OMAP_clb_TurnLightsCommand_Switch
  Constant32 : Constant  Value=OMAP_clb_JAFaultSt_Switch
  Constant33 : Constant  Value=OMAP_clb_ACCHeadwayDisplay_Switch
  Constant34 : Constant  Value=OMAP_clb_ACCHeadwayIcon_Switch
  Constant35 : Constant  Value=OMAP_clb_ACCSetSpeed_Switch
  Constant36 : Constant  Value=OMAP_clb_ACCSetSpeedDis_Switch
  Constant37 : Constant  Value=OMAP_clb_ACCStatusIconDis_Switch
  Constant38 : Constant  Value=OMAP_clb_ACC_RVVReqType_Switch
  Constant39 : Constant  Value=OMAP_clb_ACCMessagePrompt_Switch
  Constant4 : Constant  Value=OMAP_clb_DecelerationSet_Switch
  Constant40 : Constant  Value=OMAP_clb_AEBAlertReq_Switch
  Constant41 : Constant  Value=OMAP_clb_AEBFaultStatus_Switch
  Constant42 : Constant  Value=OMAP_clb_AEBSwitchStatus_Switch
  Constant43 : Constant  Value=OMAP_clb_AEBMassageDisp_Switch
  Constant44 : Constant  Value=OMAP_clb_Handsoffwarning_Switch
  Constant45 : Constant  Value=OMAP_clb_HMIPopupMassage_Switch
  Constant46 : Constant  Value=OMAP_clb_VehicleLaneDisp_Switch
  Constant47 : Constant  Value=OMAP_clb_LDWWarningSt_Switch
  Constant48 : Constant  Value=OMAP_clb_LDWStatusDisplay_Switch
  Constant49 : Constant  Value=OMAP_clb_LKAMode_Switch
  Constant5 : Constant  Value=OMAP_clb_DeclControlReq_Switch
  Constant50 : Constant  Value=OMAP_clb_LKAStatusDisplay_Switch
  Constant51 : Constant  Value=OMAP_clb_LKASwitchState_Switch
  Constant52 : Constant  Value=OMAP_clb_ELKSts_Switch
  Constant53 : Constant  Value=OMAP_clb_ICAMassageDisp_Switch
  Constant54 : Constant  Value=OMAP_clb_ICAStatusIcon_Switch
  Constant55 : Constant  Value=OMAP_clb_LCAStatusDisplay_Switch
  Constant56 : Constant  Value=OMAP_clb_LCAPopupMessage_Switch
  Constant57 : Constant  Value=OMAP_clb_ADAS_State_Switch
  Constant6 : Constant  Value=OMAP_clb_PrefillRequest_Switch
  Constant7 : Constant  Value=OMAP_clb_ESCDriveOff_Switch
  Constant8 : Constant  Value=OMAP_clb_ESCHoldReq_Switch
  Constant9 : Constant  Value=OMAP_clb_DecelerationType_Switch
  tag scope: ClbBus=global
  wires:
  Constant/1 -> Bus Creator/1  "OMAP_clb_ACCTorqueReq_Switch"
  Constant1/1 -> Bus Creator/2  "OMAP_clb_TorqueActivReq_Switch"
  Constant2/1 -> Bus Creator/3  "OMAP_clb_DownorUpGearMinTime_Switch"
  Constant3/1 -> Bus Creator/4  "OMAP_clb_ACCState_Switch"
  Constant4/1 -> Bus Creator/5  "OMAP_clb_DecelerationSet_Switch"
  Constant5/1 -> Bus Creator/6  "OMAP_clb_DeclControlReq_Switch"
  Constant6/1 -> Bus Creator/7  "OMAP_clb_PrefillRequest_Switch"
  Constant7/1 -> Bus Creator/8  "OMAP_clb_ESCDriveOff_Switch"
  Constant8/1 -> Bus Creator/9  "OMAP_clb_ESCHoldReq_Switch"
  Constant9/1 -> Bus Creator/10  "OMAP_clb_DecelerationType_Switch"
  Constant10/1 -> Bus Creator/11  "OMAP_clb_AEBState_Switch"
  Constant11/1 -> Bus Creator/12  "OMAP_clb_BrakeRequest_Switch"
  Constant12/1 -> Bus Creator/13  "OMAP_clb_AEBBrakingProg_Switch"
  Constant13/1 -> Bus Creator/14  "OMAP_clb_HapticAlarmReq_Switch"
  Constant14/1 -> Bus Creator/15  "OMAP_clb_ACCRequestEPB_Switch"
  Constant15/1 -> Bus Creator/16  "OMAP_clb_LKAState_Switch"
  Constant16/1 -> Bus Creator/17  "OMAP_clb_LKATorqFactReq_Switch"
  Constant17/1 -> Bus Creator/18  "OMAP_clb_LKAAngleReq_Switch"
  Constant18/1 -> Bus Creator/19  "OMAP_clb_LKAActivation_Switch"
  Constant19/1 -> Bus Creator/20  "OMAP_clb_ESAState_Switch"
  Constant20/1 -> Bus Creator/21  "OMAP_clb_ESATorqueReq_Switch"
  Constant21/1 -> Bus Creator/22  "OMAP_clb_ESARequest_Switch"
  Constant22/1 -> Bus Creator/23  "OMAP_clb_UpDownGearChange_Switch"
  Constant23/1 -> Bus Creator/24  "OMAP_clb_ELKPopupMessage_Switch"
  Constant24/1 -> Bus Creator/25  "OMAP_clb_ESAFaultSt_Switch"
  Constant25/1 -> Bus Creator/26  "OMAP_clb_HWAMode_Switch"
  Constant26/1 -> Bus Creator/27  "OMAP_clb_HWATurnOnIdctr_Switch"
  Constant27/1 -> Bus Creator/28  "OMAP_clb_HWAActionSts_Switch"
  Constant28/1 -> Bus Creator/29  "OMAP_clb_LightControlValid_Switch"
  Constant29/1 -> Bus Creator/30  "OMAP_clb_ISLCState_Switch"
  Constant30/1 -> Bus Creator/31  "OMAP_clb_ISLCDriverRemind_Switch"
  Constant31/1 -> Bus Creator/32  "OMAP_clb_TurnLightsCommand_Switch"
  Constant32/1 -> Bus Creator/33  "OMAP_clb_JAFaultSt_Switch"
  Constant33/1 -> Bus Creator/34  "OMAP_clb_ACCHeadwayDisplay_Switch"
  Constant34/1 -> Bus Creator/35  "OMAP_clb_ACCHeadwayIcon_Switch"
  Constant35/1 -> Bus Creator/36  "OMAP_clb_ACCSetSpeed_Switch"
  Constant36/1 -> Bus Creator/37  "OMAP_clb_ACCSetSpeedDis_Switch"
  Constant37/1 -> Bus Creator/38  "OMAP_clb_ACCStatusIconDis_Switch"
  Constant38/1 -> Bus Creator/39  "OMAP_clb_ACC_RVVReqType_Switch"
  Constant39/1 -> Bus Creator/40  "OMAP_clb_ACCMessagePrompt_Switch"
  Constant40/1 -> Bus Creator/41  "OMAP_clb_AEBAlertReq_Switch"
  Constant41/1 -> Bus Creator/42  "OMAP_clb_AEBFaultStatus_Switch"
  Constant42/1 -> Bus Creator/43  "OMAP_clb_AEBSwitchStatus_Switch"
  Constant43/1 -> Bus Creator/44  "OMAP_clb_AEBMassageDisp_Switch"
  Constant44/1 -> Bus Creator/45  "OMAP_clb_Handsoffwarning_Switch"
  Constant45/1 -> Bus Creator/46  "OMAP_clb_HMIPopupMassage_Switch"
  Constant46/1 -> Bus Creator/47  "OMAP_clb_VehicleLaneDisp_Switch"
  Constant47/1 -> Bus Creator/48  "OMAP_clb_LDWWarningSt_Switch"
  Constant48/1 -> Bus Creator/49  "OMAP_clb_LDWStatusDisplay_Switch"
  Constant49/1 -> Bus Creator/50  "OMAP_clb_LKAMode_Switch"
  Constant50/1 -> Bus Creator/51  "OMAP_clb_LKAStatusDisplay_Switch"
  Constant51/1 -> Bus Creator/52  "OMAP_clb_LKASwitchState_Switch"
  Constant52/1 -> Bus Creator/53  "OMAP_clb_ELKSts_Switch"
  Constant53/1 -> Bus Creator/54  "OMAP_clb_ICAMassageDisp_Switch"
  Constant54/1 -> Bus Creator/55  "OMAP_clb_ICAStatusIcon_Switch"
  Constant55/1 -> Bus Creator/56  "OMAP_clb_LCAStatusDisplay_Switch"
  Constant56/1 -> Bus Creator/57  "OMAP_clb_LCAPopupMessage_Switch"
  Constant57/1 -> Bus Creator/58  "OMAP_clb_ADAS_State_Switch"
  Bus Creator/1 -> [ClbBus]

== system OMAP/Runnable_OMAP_10ms_sys/OMAP_Module/Default_EMS ==
  Bus Creator : BusCreator  Inputs=7
  OMAPve_g_ACCTqReqNum : Constant  Value=-4000  OutDataTypeStr=single
  OMAPve_g_PotACCTqReqNum : Constant  Value=-4000  OutDataTypeStr=single
  OMAPve_g_TminUp_or_downGearNum : Constant  Value=0  OutDataTypeStr=single
  OMAPve_y_ACC_Engine_Start_RequestNum : Constant  Value=0  OutDataTypeStr=uint8
  OMAPve_y_Function_Acc_statusNum : Constant  Value=3  OutDataTypeStr=uint8
  OMAPve_y_Powertrain_torquewheel_requestNum : Constant  Value=0  OutDataTypeStr=uint8
  OMAPve_y_stAcvTqWhlPTPotReqNum : Constant  Value=0  OutDataTypeStr=uint8
  Default_EMS : Outport
  wires:
  OMAPve_y_ACC_Engine_Start_RequestNum/1 -> Bus Creator/1  "OMAPve_y_ACC_Engine_Start_Request_1"
  OMAPve_y_Function_Acc_statusNum/1 -> Bus Creator/7  "OMAPve_y_Function_Acc_status_1"
  OMAPve_y_stAcvTqWhlPTPotReqNum/1 -> Bus Creator/6  "OMAPve_y_stAcvTqWhlPTPotReq_1"
  OMAPve_y_Powertrain_torquewheel_requestNum/1 -> Bus Creator/4  "OMAPve_y_Powertrain_torquewheel_request_1"
  Bus Creator/1 -> Default_EMS/1  "Default_EMS"
  OMAPve_g_ACCTqReqNum/1 -> Bus Creator/3  "OMAPve_g_ACCTqReq_1"
  OMAPve_g_PotACCTqReqNum/1 -> Bus Creator/2  "OMAPve_g_PotACCTqReq_1"
  OMAPve_g_TminUp_or_downGearNum/1 -> Bus Creator/5  "OMAPve_g_TminUp_or_downGear_1"

== system OMAP/Runnable_OMAP_10ms_sys/OMAP_Module/Default_EPS ==
  Bus Creator10 : BusCreator  Inputs=8
  Constant : Constant  Value=0  OutDataTypeStr=uint8
  Constant1 : Constant  Value=0  OutDataTypeStr=single
  Constant2 : Constant  Value=0  OutDataTypeStr=uint8
  OMAPve_g_Coefficient_toregulate_EPSNum : Constant  Value=0  OutDataTypeStr=single
  OMAPve_g_Column_angle_setpoint3F2Num : Constant  Value=0  OutDataTypeStr=single
  OMAPve_y_General_state_of_LKA_function3F2Num : Constant  Value=0  OutDataTypeStr=uint8
  OMAPve_y_Permit_to_know_if_LKA_or_LPA3F2Num : Constant  Value=0  OutDataTypeStr=uint8
  OMAPve_y_Power_steering_power_cut3F2Num : Constant  Value=0  OutDataTypeStr=uint8
  Default_EPS : Outport
  wires:
  OMAPve_y_Power_steering_power_cut3F2Num/1 -> Bus Creator10/1  "OMAPve_y_Power_steering_power_cut3F2_2"
  OMAPve_y_General_state_of_LKA_function3F2Num/1 -> Bus Creator10/2  "OMAPve_y_General_state_of_LKA_function3F2_2"
  Bus Creator10/1 -> Default_EPS/1  "Default_EPS"
  OMAPve_g_Coefficient_toregulate_EPSNum/1 -> Bus Creator10/3  "OMAPve_g_Coefficient_toregulate_EPS_2"
  OMAPve_y_Permit_to_know_if_LKA_or_LPA3F2Num/1 -> Bus Creator10/5  "OMAPve_y_Permit_to_know_if_LKA_or_LPA3F2_2"
  OMAPve_g_Column_angle_setpoint3F2Num/1 -> Bus Creator10/4  "OMAPve_g_Column_angle_setpoint3F2_2"
  Constant1/1 -> Bus Creator10/7  "OMAPve_g_ADAS_ESATorqueReq_2"
  Constant/1 -> Bus Creator10/6  "OMAPve_y_ADAS_ESAState_2"
  Constant2/1 -> Bus Creator10/8  "OMAPve_y_ADAS_ESARequest_2"

== system OMAP/Runnable_OMAP_10ms_sys/OMAP_Module/Default_ESC ==
  Bus Creator5 : BusCreator  Inputs=13
  OMAPve_g_Deceleration_setpoint_deviceNum : Constant  Value=2.05  OutDataTypeStr=single
  OMAPve_y_ADAS_ACCRequestEPBNum : Constant  Value=0  OutDataTypeStr=uint8
  OMAPve_y_ADAS_ESCDriveOffNum : Constant  Value=0  OutDataTypeStr=uint8
  OMAPve_y_ADAS_ESCHoldReqNum : Constant  Value=0  OutDataTypeStr=uint8
  OMAPve_y_AEB_Braking_progressNum : Constant  Value=0  OutDataTypeStr=uint8
  OMAPve_y_AEB_StatusNum : Constant  Value=0  OutDataTypeStr=uint8
  OMAPve_y_Decel_RequestNum : Constant  Value=0  OutDataTypeStr=uint8
  OMAPve_y_FCW_StatusNum : Constant  Value=10  OutDataTypeStr=uint8
  OMAPve_y_Haptic_AlarmNum : Constant  Value=0  OutDataTypeStr=uint8
  OMAPve_y_MDD_Decelerationcontrol_requestNum : Constant  Value=0  OutDataTypeStr=uint8
  OMAPve_y_MDD_deceleration_typeNum : Constant  Value=0  OutDataTypeStr=uint8
  OMAPve_y_Prefill_requestNum : Constant  Value=0  OutDataTypeStr=uint8
  OMAPve_y_State_of_the_functionFARC_detNum : Constant  Value=0  OutDataTypeStr=uint8
  Default_ESC : Outport
  wires:
  OMAPve_g_Deceleration_setpoint_deviceNum/1 -> Bus Creator5/8  "OMAPve_g_Deceleration_setpoint_device_1"
  OMAPve_y_FCW_StatusNum/1 -> Bus Creator5/1  "OMAPve_y_FCW_Status_1"
  OMAPve_y_Haptic_AlarmNum/1 -> Bus Creator5/5  "OMAPve_y_Haptic_Alarm_1"
  OMAPve_y_State_of_the_functionFARC_detNum/1 -> Bus Creator5/2  "OMAPve_y_State_of_the_functionFARC_det_1"
  OMAPve_y_AEB_Braking_progressNum/1 -> Bus Creator5/12  "OMAPve_y_AEB_Braking_progress_1"
  OMAPve_y_Decel_RequestNum/1 -> Bus Creator5/11  "OMAPve_y_Decel_Request_1"
  OMAPve_y_MDD_deceleration_typeNum/1 -> Bus Creator5/10  "OMAPve_y_MDD_deceleration_type_1"
  OMAPve_y_AEB_StatusNum/1 -> Bus Creator5/3  "OMAPve_y_AEB_Status_1"
  Bus Creator5/1 -> Default_ESC/1  "Default_ESC"
  OMAPve_y_Prefill_requestNum/1 -> Bus Creator5/4  "OMAPve_y_Prefill_request_1"
  OMAPve_y_MDD_Decelerationcontrol_requestNum/1 -> Bus Creator5/9  "OMAPve_y_MDD_Decelerationcontrol_request_1"
  OMAPve_y_ADAS_ESCDriveOffNum/1 -> Bus Creator5/6  "OMAPve_y_ADAS_ESCDriveOff"
  OMAPve_y_ADAS_ESCHoldReqNum/1 -> Bus Creator5/7  "OMAPve_y_ADAS_ESCHoldReq"
  OMAPve_y_ADAS_ACCRequestEPBNum/1 -> Bus Creator5/13  "OMAPve_y_ADAS_ACCRequestEPB"
